simulink model "ejemploDB"  (R2018a)
settings: Solver=VariableStepAuto  StartTime=0.0  StopTime=10.0  RelTol=1e-3
settings Model: Creator=carma  LastModifiedBy=carma

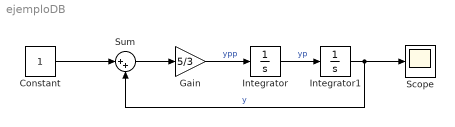
== system ejemploDB ==
  Constant : Constant
  Gain : Gain  Gain=5/3
  Integrator : Integrator
  Integrator1 : Integrator
  Scope : Scope
  Sum : Sum  Inputs=|++
  wires:
  Sum/1 -> Gain/1
  Constant/1 -> Sum/1
  Integrator1/1 -> Scope/1, Sum/2  "y"
  Gain/1 -> Integrator/1  "ypp"
  Integrator/1 -> Integrator1/1  "yp"
